simulink model "DummyVehicleModel_2019b"  (R2019b)
settings: Solver=FixedStepAuto  StartTime=0.0  StopTime=200  FixedStep=0.001  RelTol=1e-3
values from neighbouring files (symbols this model uses):
  RealSimPara = struct    [ecodrivingMain.m]
settings Model: Creator=y0n  LastModifiedBy=hg25079
settings DataIOCC: SaveOutput=off  SignalLogging=off  DSMLogging=off  SaveTime=off  ReturnWorkspaceOutputsName=VehicleOut
settings DebuggingCC: AlgebraicLoopMsg=none  UnderSpecifiedDimensionMsg=error
settings SFSimCC: CustomCodeUndefinedFunction=UseInterfaceOnly

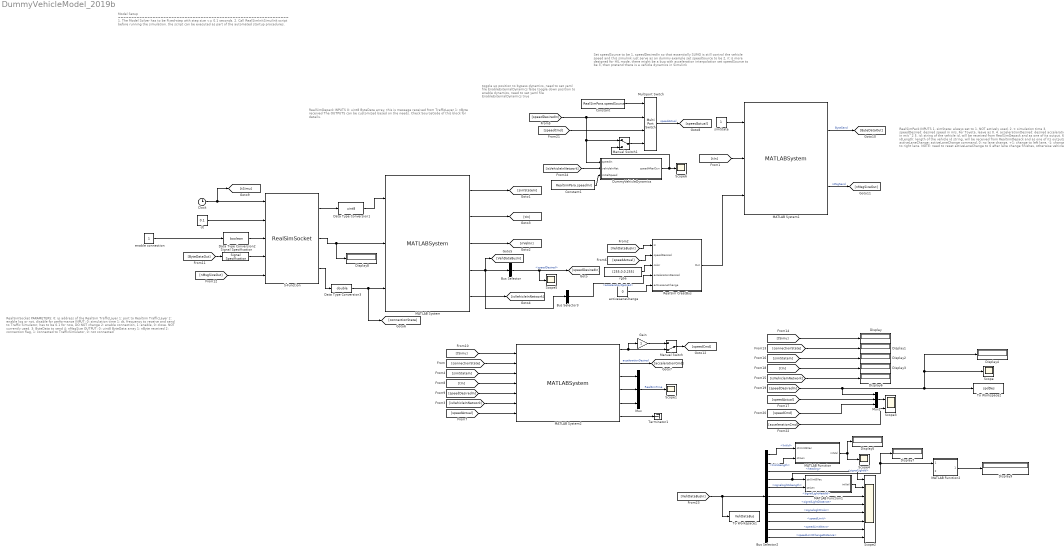
== system DummyVehicleModel_2019b ==
  note: toggle up position to bypass dynamics, need to set yaml file EnableExternalDynamics false
      | toggle down position to enable dynamics, need to set yaml file EnableExternalDynamics true
  note: Set speedSource to be 1, speedDesiredIn so that essentially SUMO is still control the vehicle speed and this simulink just serve as an dummy example
      |
      | set speedSource to be 2, it is more designed for HIL mode, there might be a bug with acceleration interpolation
      |
      | set speedSource to be 3, then pretend there is a vehicle dynamics in Simulink
  note: Model Setup
      | ================================================================
      | 1. The Model Solver has to be Fixed-step with step size <= 0.1 seconds.
      | 2. Call RealSimInitSimulink script before running the simulation. the script can be executed as part of the automated startup procedures.
  note: RealSimSocket
      | PARAMETERS:
      | 0: ip address of the RealSim TrafficLayer
      | 1: port to RealSim TrafficLayer
      | 2: enable log or not, disable for performance
      | INPUT:
      | 0: simulation time
      | 1: dt, frequency to receive and send to Traffic Simulator, has to be 0.1 for now, DO NOT change
      | 2: enable connection, 1: enable, 0: close. NOT currently used.
      | 3: ByteData to send
      | 4: nMsgSize
      |
      | OUTPUT:
      | 0: uint8 ByteData array
      | 1: nByte received
      | 2: connection flag, 1: connected to TrafficSimulator, 0: not connected
  note: RealSimPack
      | INPUTS
      | 1. simState: always set to 1. NOT actively used.
      | 2. t: simulation time
      | 3. speedDesired: desired speed in m/s, For Toyota, leave as 0.
      | 4. accelerationDesired: desired acceleration in m/s^2
      | 5. id: string of the vehicle id, will be received from RealSimDepack and as one of its output.
      | 6. idLength: length of the vehicle id string, will be received from RealSimDepack and as one of its outputs
      | 7: activeLaneChange: activeLaneChange command, 0: no lane change, +1: change to left lane, -1: change to right lane. NOTE: need to reset activeLaneChange to 0 after lane change finishes, otherwise vehicle will keep making lane change. Will receive 0 activeLaneChangeFdbk from RealSimDepack when lane change finishes.
      |
      | NOTE 1: Currently, only speedDesired and/or accelerationDesired can be sent to VISSIM/SUMO. The data format receive and send are the same so other mesage fields of the send data are irrelevant and can be set to empty or zero.
      |
      | NOTE 2: if select both speedDesired and accelerationDesired
      | in config.yaml, then only accelerationDesired will be used
      | to control vehicles in TrafficSimulator. if only one of
      | speedDesired and accelerationDesired selected in
      | config.yaml, then the one selected will be used for
      | control, the other input can be leave as 0.
      |
      | NOTE 3: for VISSIM, speedDesired or accelerationDesired will be the control command 0.2 seconds in the future.
      |
      | OUTPUTS
      | 1.ByteData: bytes vector that will be sent to TrafficSimualtor
      | 2.nMsgSize: size of bytes to be sent
  note: RealSimDepack
      | INPUTS
      | 0: uint8 ByteData array, this is message received from TrafficLayer
      | 1: nByte received
      |
      | The OUTPUTS can be customized based on the needs. Check SourceCode of this block for details.
  Bus Selector : BusSelector  OutputSignals=speedDesired
  Bus Selector2 : BusSelector  OutputSignals=linkId,linkIdLength,heading,signalLightId,signalLightIdLength,signalLightHeadId,signalLightDistance,signalLightColor,speedLimit,speedLimitNext,speedLimitChangeDistance
  Bus Selector3 : BusSelector  OutputSignals=accelerationDesired
  Clock : Clock
  Constant : Constant  Value=RealSimPara.speedSource
  Constant1 : Constant  Value=RealSimPara.speedInit
  Data Type Conversion1 : DataTypeConversion  OutDataTypeStr=uint8
  Data Type Conversion2 : DataTypeConversion  OutDataTypeStr=boolean
  Data Type Conversion3 : DataTypeConversion  OutDataTypeStr=double
  Display{,1..9} (10 alike) : Display
  DummyVehicleDynamics : Subsystem
  Gain : Gain
  MATLAB Function : MATLAB Function  TreatAsAtomicUnit=on
  MATLAB Function1 : MATLAB Function  TreatAsAtomicUnit=on
  MATLAB Function2 : MATLAB Function  TreatAsAtomicUnit=on  SystemSampleTime=0.001
  MATLAB System : MATLABSystem  System=RealSimDepack  OutputBusName=VehDataBus  VehicleMessageFieldDefInputVec=VehicleMessageFieldDefInputVec  SimulateUsing=Code generation
      mask Type: RealSimDepack
      mask Display:
      | disp('RealSimDepack');
      | port_label('input',1,'ByteData');
      | port_label('input',2,'nByte');
      | port_label('input',3,'connectionState');
      | port_label('output',1,'simState');
      | port_label('output',2,'t');
      | port_label('output',3,'nVeh');
      | port_label('output',4,'VehDataBus');
      | port_label('output',5,'isVehicleInNetwork');
  MATLAB System1 : MATLABSystem  System=RealSimPack  VehicleMessageFieldDefInputVec=VehicleMessageFieldDefInputVec  SimulateUsing=Code generation
      mask Type: RealSimPack
      mask Display:
      | disp('RealSimPack');
      | port_label('input',1,'simState');
      | port_label('input',2,'t');
      | port_label('input',3,'VehDataBus');
      | port_label('output',1,'ByteData');
      | port_label('output',2,'nMsgSize');
  MATLAB System2 : MATLABSystem  System=RealSimInterpSpeed  initialSpeed=RealSimPara.speedInit  speedLookAheadHorizon=RealSimPara.tLookahead  speedUpperBound=30  smoothWindow=RealSimPara.smoothWindow  SimulateUsing=Code generation
      mask Type: RealSimInterpSpeed
      mask Display:
      | disp('RealSimInterpSpeed');
      | port_label('input',1,'simulationTime');
      | port_label('input',2,'connectionState');
      | port_label('input',3,'simState');
      | port_label('input',4,'timeReceive');
      | port_label('input',5,'speedReceive');
      | port_label('input',6,'isVehicleInNetwork');
      | port_label('input',7,'speedActual');
      | port_label('output',1,'speedLookAhead');
      | port_label('output',2,'accelerationDesired');
      | port_label('output',3,'timeSimulator');
      | port_label('output',4,'timeStepSimulator');
      | port_label('output',5,'timeStepTrigger');
      | port_label('output',6,'RealSimDelay');
  Manual Switch : ManualSwitch  CurrentSetting=0
  Manual Switch1 : ManualSwitch
  Multiport Switch : MultiPortSwitch
  Mux : Mux  Inputs=3
  Mux1 : Mux  Inputs=3
  RealSim CreatBus : Subsystem
  S-Function : S-Function  FunctionName=RealSimSocket  Parameters=TrafficLayerIP, TrafficLayerPort, 0  SFunctionDeploymentMode=off  EnableBusSupport=off
  Scope{,1,4..6} (5 alike) : Scope
  Scope2 : Scope  NumInputPorts=8
  Scope3 : Scope  NumInputPorts=2
  Signal Specification : SignalSpecification  Dimensions=[200 1]
  Terminator1 : Terminator
  To Workspace1 : ToWorkspace  VariableName=VehDataBus  SaveFormat=Timeseries  SampleTime=-1
  To Workspace2 : ToWorkspace  VariableName=spdDes  SaveFormat=Structure With Time  SampleTime=-1
  activeLaneChange : Constant  Value=0
  dt : Constant  Value=0.1
  enable connection : Constant
  rgba : Constant  Value=[255,0,0,255]
  simState : Constant
  wires:
  dt/1 -> S-Function/2
  S-Function/1 -> Data Type Conversion1/1
  S-Function/2 -> Display8/1, MATLAB System/2
  Data Type Conversion1/1 -> MATLAB System/1
  enable connection/1 -> Data Type Conversion2/1
  Data Type Conversion2/1 -> S-Function/3
  S-Function/3 -> Data Type Conversion3/1
  MATLAB System/1 -> [simStateIn]
  Signal Specification/1 -> S-Function/4
  Bus Selector/1 -> Scope5/1, [speedDesiredIn]  "<speedDesired>"
  MATLAB System/2 -> [tIn]
  MATLAB System/3 -> [nVehIn]
  MATLAB System/5 -> [isVehicleInNetwork]
  Data Type Conversion3/1 -> [connectionState], MATLAB System/3
  MATLAB System/4 -> Bus Selector3/1, [VehDataBusIn], Bus Selector/1
  [speedDesiredIn] -> MATLAB System2/5
  [tIn] -> MATLAB System2/4
  [connectionState] -> MATLAB System2/2
  [isVehicleInNetwork] -> MATLAB System2/6
  [simStateIn] -> MATLAB System2/3
  [tSimu] -> MATLAB System2/1
  Multiport Switch/1 -> [speedActual]  "speedActual"
  [speedActual] -> MATLAB System2/7
  Clock/1 -> [tSimu], S-Function/1
  [ByteDataOut] -> Signal Specification/1
  [nMsgSizeOut] -> S-Function/5
  MATLAB System2/1 -> Gain/1, Manual Switch/2
  MATLAB System2/2 -> [accelerationCmd]  "accelerationDesired"
  MATLAB System2/3 -> Mux/1
  MATLAB System2/4 -> Mux/2
  MATLAB System2/5 -> Mux/3
  Mux/1 -> Scope1/1  "RealSimTime"
  MATLAB System2/6 -> Terminator1/1
  rgba/1 -> RealSim CreatBus/3(color)
  [tIn] -> MATLAB System1/2
  RealSim CreatBus/1(Out) -> MATLAB System1/3
  [speedActual] -> RealSim CreatBus/2(speedDesired)
  MATLAB System1/2 -> [nMsgSizeOut]  "nMsgSend"
  MATLAB System1/1 -> [ByteDataOut]  "ByteSend"
  simState/1 -> MATLAB System1/1
  [VehDataBusIn] -> RealSim CreatBus/1(In)
  [accelerationCmd] -> Scope3/2
  Mux1/1 -> Scope3/1
  [speedActual] -> Mux1/2
  [tSimu] -> Display/1
  [speedDesiredIn] -> Display4/1, Scope/1, To Workspace2/1, Mux1/1
  [speedCmd] -> Mux1/3
  [connectionState] -> Display1/1
  [tIn] -> Display3/1
  [simStateIn] -> Display2/1
  [isVehicleInNetwork] -> Display6/1
  [speedDesiredIn] -> Multiport Switch/2, DummyVehicleDynamics/1(speedIn), Manual Switch1/1
  activeLaneChange/1 -> RealSim CreatBus/5(activeLaneChange)
  Bus Selector3/1 -> RealSim CreatBus/4(accelerationDesired)  "<accelerationDesired>"
  Constant/1 -> Multiport Switch/1
  Manual Switch1/1 -> Multiport Switch/4
  [speedCmd] -> Multiport Switch/3
  Bus Selector2/8 -> Scope2/5  "<signalLightColor>"
  Bus Selector2/5 -> MATLAB Function1/2(strLen)  "<signalLightIdLength>"
  Bus Selector2/4 -> MATLAB Function2/1(signalLightId), Display7/1, MATLAB Function1/1(strUint8Vec)  "<signalLightId>"
  MATLAB Function/1(intVal) -> Scope4/1, Display5/1
  Bus Selector2/9 -> Scope2/6  "<speedLimit>"
  Bus Selector2/7 -> Scope2/4  "<signalLightDistance>"
  Bus Selector2/1 -> MATLAB Function/1(strUint8Vec)  "<linkId>"
  Bus Selector2/10 -> Scope2/7  "<speedLimitNext>"
  Bus Selector2/2 -> MATLAB Function/2(strLen)  "<linkIdLength>"
  Bus Selector2/11 -> Scope2/8  "<speedLimitChangeDistance>"
  Bus Selector2/3 -> Scope2/1  "<heading>"
  Bus Selector2/6 -> Scope2/3  "<signalLightHeadId>"
  [VehDataBusIn] -> To Workspace1/1, Bus Selector2/1
  MATLAB Function1/1(intVal) -> Scope2/2
  MATLAB Function2/1(signalLightIdString) -> Display9/1
  Manual Switch/1 -> [speedCmd]
  Gain/1 -> Manual Switch/1
  DummyVehicleDynamics/1(speedAfterDyn) -> Scope6/1, Manual Switch1/2
  [isVehicleInNetwork] -> DummyVehicleDynamics/2(vehicleInNet)
  Constant1/1 -> DummyVehicleDynamics/3(initialSpeed)

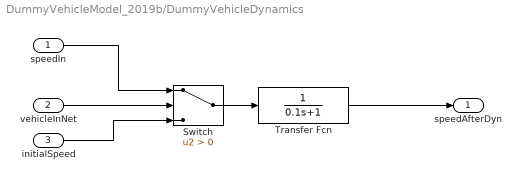
== system DummyVehicleModel_2019b/DummyVehicleDynamics ==
  speedIn : Inport
  vehicleInNet : Inport  Port=2
  initialSpeed : Inport  Port=3
  Switch : Switch  Criteria=u2 > Threshold
  Transfer Fcn : TransferFcn  Denominator=[0.1 1]
  speedAfterDyn : Outport
  wires:
  Transfer Fcn/1 -> speedAfterDyn/1
  speedIn/1 -> Switch/1
  vehicleInNet/1 -> Switch/2
  initialSpeed/1 -> Switch/3
  Switch/1 -> Transfer Fcn/1

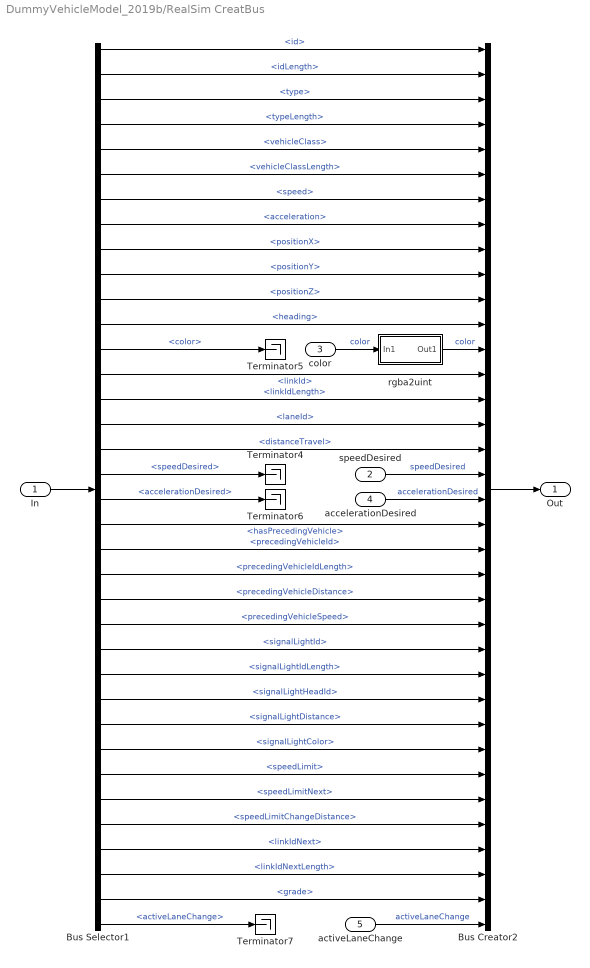
== system DummyVehicleModel_2019b/RealSim CreatBus ==
  In : Inport
  speedDesired : Inport  Port=2
  color : Inport  Port=3
  accelerationDesired : Inport  Port=4
  activeLaneChange : Inport  Port=5
  Bus Creator2 : BusCreator  Inputs=36  OutDataTypeStr=Bus: VehDataBus
  Bus Selector1 : BusSelector  OutputSignals=id,idLength,type,typeLength,vehicleClass,vehicleClassLength,speed,acceleration,positionX,positionY,positionZ,heading,color,linkId,linkIdLength,laneId,distanceTravel,speedDesired,accelerationDesired,hasPrecedingVehicle,precedingVehicleId,precedingVehicleIdLength,precedingVehicleDistance,precedingVehicleSpeed,signalLightId,signalLightIdLength,signalLightHeadId,signalLightDistance,signalLightColor,speedLimit,speedLimitNext,speedLimitChangeDistance,linkIdNext,linkIdNextLength,grade,activeLaneChange
  Terminator{4..7} (4 alike) : Terminator
  rgba2uint : Subsystem
  Out : Outport
  wires:
  In/1 -> Bus Selector1/1
  Bus Selector1/1 -> Bus Creator2/1  "<id>"
  Bus Selector1/2 -> Bus Creator2/2  "<idLength>"
  Bus Selector1/3 -> Bus Creator2/3  "<type>"
  Bus Selector1/4 -> Bus Creator2/4  "<typeLength>"
  Bus Selector1/5 -> Bus Creator2/5  "<vehicleClass>"
  Bus Selector1/6 -> Bus Creator2/6  "<vehicleClassLength>"
  Bus Selector1/7 -> Bus Creator2/7  "<speed>"
  Bus Selector1/8 -> Bus Creator2/8  "<acceleration>"
  Bus Selector1/9 -> Bus Creator2/9  "<positionX>"
  Bus Selector1/10 -> Bus Creator2/10  "<positionY>"
  Bus Selector1/11 -> Bus Creator2/11  "<positionZ>"
  Bus Selector1/12 -> Bus Creator2/12  "<heading>"
  Bus Selector1/13 -> Terminator5/1  "<color>"
  Bus Selector1/14 -> Bus Creator2/14  "<linkId>"
  Bus Selector1/15 -> Bus Creator2/15  "<linkIdLength>"
  Bus Selector1/16 -> Bus Creator2/16  "<laneId>"
  Bus Selector1/17 -> Bus Creator2/17  "<distanceTravel>"
  Bus Selector1/18 -> Terminator4/1  "<speedDesired>"
  Bus Selector1/19 -> Terminator6/1  "<accelerationDesired>"
  Bus Selector1/20 -> Bus Creator2/20  "<hasPrecedingVehicle>"
  Bus Selector1/21 -> Bus Creator2/21  "<precedingVehicleId>"
  Bus Selector1/22 -> Bus Creator2/22  "<precedingVehicleIdLength>"
  Bus Selector1/23 -> Bus Creator2/23  "<precedingVehicleDistance>"
  Bus Selector1/24 -> Bus Creator2/24  "<precedingVehicleSpeed>"
  Bus Selector1/25 -> Bus Creator2/25  "<signalLightId>"
  Bus Selector1/26 -> Bus Creator2/26  "<signalLightIdLength>"
  Bus Selector1/27 -> Bus Creator2/27  "<signalLightHeadId>"
  Bus Selector1/28 -> Bus Creator2/28  "<signalLightDistance>"
  Bus Selector1/29 -> Bus Creator2/29  "<signalLightColor>"
  Bus Selector1/30 -> Bus Creator2/30  "<speedLimit>"
  Bus Selector1/31 -> Bus Creator2/31  "<speedLimitNext>"
  Bus Selector1/32 -> Bus Creator2/32  "<speedLimitChangeDistance>"
  Bus Selector1/33 -> Bus Creator2/33  "<linkIdNext>"
  Bus Selector1/34 -> Bus Creator2/34  "<linkIdNextLength>"
  Bus Selector1/35 -> Bus Creator2/35  "<grade>"
  Bus Selector1/36 -> Terminator7/1  "<activeLaneChange>"
  activeLaneChange/1 -> Bus Creator2/36  "activeLaneChange"
  speedDesired/1 -> Bus Creator2/18  "speedDesired"
  accelerationDesired/1 -> Bus Creator2/19  "accelerationDesired"
  color/1 -> rgba2uint/1(In1)  "color"
  rgba2uint/1(Out1) -> Bus Creator2/13  "color"
  Bus Creator2/1 -> Out/1

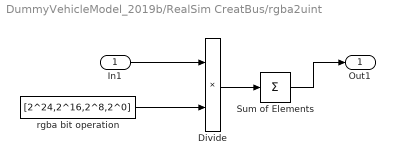
== system DummyVehicleModel_2019b/RealSim CreatBus/rgba2uint ==
  In1 : Inport
  Divide : Product  Inputs=**
  Sum of Elements : Sum  Inputs=+
  rgba bit operation : Constant  Value=[2^24,2^16,2^8,2^0]
  Out1 : Outport
  wires:
  Divide/1 -> Sum of Elements/1
  In1/1 -> Divide/1
  rgba bit operation/1 -> Divide/2
  Sum of Elements/1 -> Out1/1

== matlab function DummyVehicleModel_2019b/MATLAB Function1 ==
  data: strUint8Vec input; intVal output double; strLen input
function intVal = strVec2Int(strUint8Vec, strLen)

    strVec = blanks(50);
    for i = 1:strLen
       strVec(i) = strUint8Vec(i); 
    end
    if strLen > 0
        intVal = real(str2double(strVec(1:strLen)));
    else
        intVal = -1;
    end

== matlab function DummyVehicleModel_2019b/MATLAB Function ==
  data: strUint8Vec input; intVal output double; strLen input
function intVal = strVec2Int(strUint8Vec, strLen)

    strVec = blanks(50);
    for i = 1:strLen
       strVec(i) = strUint8Vec(i); 
    end
    if strLen > 0
        intVal = real(str2double(strVec(1:strLen)));
    else
        intVal = -1;
    end

== matlab function DummyVehicleModel_2019b/MATLAB Function2 ==
  data: signalLightId input uint8 size=[1 50]; signalLightIdString output string; signalLightIdLength input
function signalLightIdString = fcn(signalLightId, signalLightIdLength)

signalLightIdString = string(char(signalLightId));
